simulink model "Postoian"  (R2019a)
settings: Solver=FixedStepAuto  StartTime=0.0  StopTime=1  FixedStep=0.0001  RelTol=1e-4
values from neighbouring files (symbols this model uses):
  b1 = [3.31578564644 0.905199348927 -1.07588481903 -9.39754581451 6.51989841461 -7.39431810379 -7.98054647446 -7.51470994949 -2.46217346191 -2.60606265068 0.634998142719 -7.34759140015 ... (20 elements, 1x20)]    [b1.mat]
  b2 = [-8.908867836 -6.37810707092 -8.66125679016 -6.19361543655 -8.59416675568 -9.12425804138 -8.47231483459 -9.20506572723 -8.79118919373 -9.36305236816 -9.80707740784 -1.32926535606 ... (15 elements, 1x15)]    [b2.mat]
  b3 = 0.566753208637    [b3.mat]
  w1 = [-3.38608121872 -1.61282348633 -0.811974227428 -26.1486988068 -5.43596601486 -2.50496292114 -2.73406887054 -1.47529745102 -13.9745950699 -4.77835845947 -8.42057037354 -10.048833847 ... (100 elements, 5x20)]    [w1.mat]    (also in w1d.mat = [-28.5484638214 -28.3087368011 -16.2038860321 -18.8476390839)
  w2 = [-1.73702144623 -0.185042783618 -1.43662083149 5.53469181061 0.114013127983 -6.10858488083 1.57797574997 1.2862662077 -7.84612417221 -0.614148855209 -15.9998350143 -5.41085386276 ... (300 elements, 20x15)]    [w2.mat]    (also in w2d.mat = [-15.8134098053 -19.7163829803 -21.1157608032 -0.21424435079)
  w3 = [0.296215087175 2.04968070984 0.382735908031 1.65471422672 0.95603877306]    [w3.mat]    (also in w3d.mat = [-2.66624140739 1.28664553165 0.95645904541 -5.20410871506 2)
libraries: simulink x2, neural x2
settings Model: NumberOfSteps=10  Creator=70810  LastModifiedBy=70810
settings SolverCC: AlgebraicLoopSolver=LineSearch

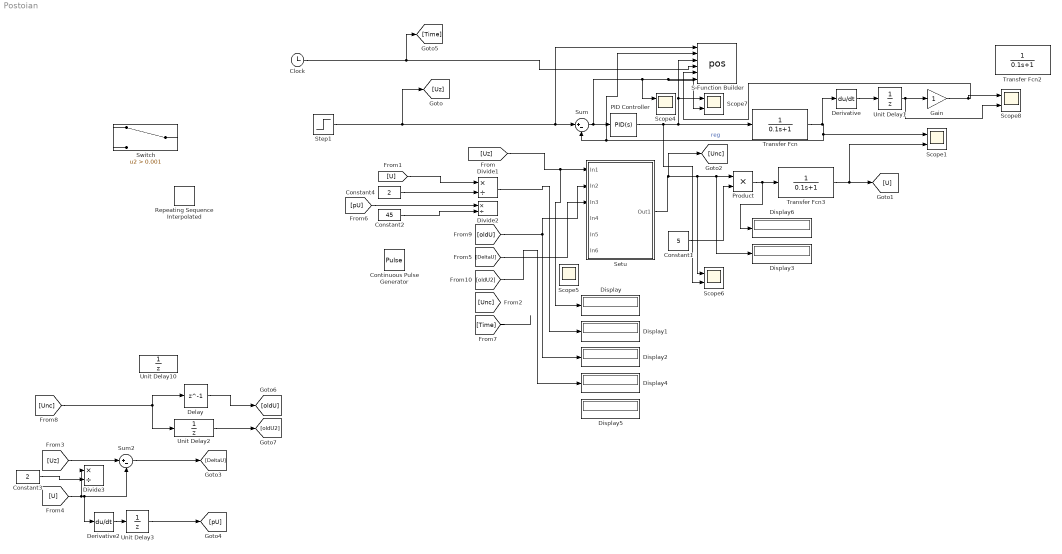
== system Postoian ==
  Clock : Clock
  Constant1 : Constant  Value=5
  Constant2 : Constant  Value=45
  Constant3 : Constant  Value=2
  Constant4 : Constant  Value=2
  Continuous Pulse Generator : DiscretePulseGenerator  PulseType=Time based  Period=1  PulseWidth=50
  Delay : Delay  DelayLength=1  InitialCondition=0
  Derivative : Derivative
  Derivative2 : Derivative
  Display{,1..6} (7 alike) : Display
  Divide1 : Product  Inputs=*/
  Divide2 : Product  Inputs=*/
  Divide3 : Product  Inputs=*/
  Gain : Gain
  PID Controller : simulink/Continuous/PID Controller  Controller=PID  Form=Parallel  TimeDomain=Continuous-time  SampleTime=-1  IntegratorMethod=Forward Euler  FilterMethod=Forward Euler  ControllerParametersSource=internal  P=4  I=255  D=0  UseFilter=on  N=100  TunerSelectOption=Transfer Function Based (PID Tuner App)  InitialConditionSource=internal  InitialConditionForIntegrator=0  InitialConditionForFilter=0  DifferentiatorICPrevScaledInput=0  ExternalReset=none  TrackingMode=off  Kt=1  LimitOutput=off  UpperSaturationLimit=inf  LowerSaturationLimit=-inf  LinearizeAsGain=on  AntiWindupMode=none  Kb=1  POutMin=[]  POutMax=[]  IOutMin=[]  IOutMax=[]  DOutMin=[]  DOutMax=[]  NOutMin=[]  NOutMax=[]  SumOutMin=[]  SumOutMax=[]  SaturationOutMin=[]  SaturationOutMax=[]  PParamMin=[]  PParamMax=[]  IParamMin=[]  IParamMax=[]  DParamMin=[]  DParamMax=[]  NParamMin=[]  NParamMax=[]  KbParamMin=[]  KbParamMax=[]  KtParamMin=[]  KtParamMax=[]  KbOutMin=[]  KbOutMax=[]  KtOutMin=[]  KtOutMax=[]  IntegratorOutMin=[]  IntegratorOutMax=[]  FilterOutMin=[]  FilterOutMax=[]  SumI1OutMin=[]  SumI1OutMax=[]  SumI2OutMin=[]  SumI2OutMax=[]  SumI3OutMin=[]  SumI3OutMax=[]  SumI4OutMin=[]  SumI4OutMax=[]  SumDOutMin=[]  SumDOutMax=[]  DifferentiatorOutMin=[]  DifferentiatorOutMax=[]  FilterDiffOutCoefMin=[]  FilterDiffOutCoefMax=[]  ReciprocalOutMin=[]  ReciprocalOutMax=[]  SumDenOutMin=[]  SumDenOutMax=[]  SumNumOutMin=[]  SumNumOutMax=[]  DivideOutMin=[]  DivideOutMax=[]  IntegratorContinuousStateAttributes=''  IntegratorStateMustResolveToSignalObject=off  IntegratorRTWStateStorageClass=Auto  FilterContinuousStateAttributes=''  FilterStateMustResolveToSignalObject=off  FilterRTWStateStorageClass=Auto  ParallelPVariant=InternalParameters  IdealPVariant=Disabled  IVariant=InternalParameters  DVariant=InternalParameters  IntegratorVariant=Continuous  SatVariant=Disabled  AWVariant=Passthrough  PCopyVariant=Disabled  TRVariant=Disabled  FdbkBlocksVariant=Forward  IdealPFdbkVariant=Disabled  SatFdbkVariant=Disabled  DerivativeFilterVariant=ContFilter  NVariant=InternalParameters  NCopyVariant=Disabled  FilterICVariant=InternalICsFilter  IntegratorICVariant=InternalICs  ExternalResetVariant=Disabled  TRSumVariant=Passthrough  SumFdbkVariant=Disabled  SumVariant=Sum_PID
  Product : Product
  Repeating Sequence Interpolated : simulink/Sources/Repeating Sequence Interpolated  OutValues=[0 0.5 1 1 0.5 0].'  TimeValues=[0 0.2 0.4 0.6 0.8 1].'  LookUpMeth=Interpolation-Use End Values  tsamp=0.01  OutMin=[]  OutMax=[]  OutDataTypeStr=double  OutputDataTypeScalingMode=double  OutDataType=fixdt(0,8)  OutScaling=2^-10
  S-Function Builder : S-Function  InitFcn=try, set_param(gcb,'FunctionName','pos'), end  FunctionName=pos  SFunctionModules=pos_wrapper Aray  SFunctionDeploymentMode=off  EnableBusSupport=off  mask(S-Function Builder){}
      mask help: Simulink:masks:SFunctionBuilder_MD
      mask init:
      | val = [[.9  0.75 0.75 1 1 .9 .9 1]',[1 1 0.75 0.75 .9 .9 1 .9]'];try , sys = get_param(gcb,'SfunBuilderFcnName');if isempty(sys), sys = get_param(gcb,'FunctionName'); end,catch, sys = get_param(gcb,'FunctionName'); end
      settings: CopyFcn=set_param(gcbh,'LinkStatus','none')  PreSaveFcn=try, set_param(gcb,'FunctionName','pos'), end  OpenFcn=sfunctionwizard(gcbh)
      mask Display: plot(val(:,1),val(:,2)),disp(sys), port_label('input',1,'u0'), port_label('input',2,'u1'), port_label('input',3,'u2'), port_label('input',4,'u3'), port_label('input',5,'u4'), port_label('input',6,'u5'), port_label('output',1,'y0')
  Scope{1,4..8} (6 alike) : Scope  NumInputPorts=2
  Setu : Subsystem
  Step1 : Step  Time=0.1  SampleTime=0
  Sum : Sum  Inputs=|+-
  Sum2 : Sum  Inputs=|+-
  Switch : Switch  Criteria=u2 > Threshold  Threshold=0.001
  Transfer Fcn : TransferFcn  Denominator=[0.1 1]
  Transfer Fcn2 : TransferFcn  Denominator=[0.1 1]
  Transfer Fcn3 : TransferFcn  Denominator=[0.1 1]
  Unit Delay1 : UnitDelay  SampleTime=0.0001  HasFrameUpgradeWarning=on
  Unit Delay10 : UnitDelay  SampleTime=0.0001  HasFrameUpgradeWarning=on
  Unit Delay2 : UnitDelay  SampleTime=0.0002  HasFrameUpgradeWarning=on
  Unit Delay3 : UnitDelay  SampleTime=0.0001  HasFrameUpgradeWarning=on
  wires:
  PID Controller/1 -> Scope6/2, Scope7/1, S-Function Builder/3, Transfer Fcn/1
  Transfer Fcn/1 -> Derivative/1, Scope1/1, Sum/2, S-Function Builder/2  "reg"
  Sum/1 -> Scope4/1, Scope7/2, S-Function Builder/6, PID Controller/1
  Product/1 -> Display6/1, Transfer Fcn3/1
  Transfer Fcn3/1 -> [U], Scope1/2
  Constant4/1 -> Divide1/2
  Constant1/1 -> Product/2
  Derivative/1 -> Unit Delay1/1
  Unit Delay1/1 -> Scope8/2, Gain/1
  Gain/1 -> Scope8/1, S-Function Builder/5
  Constant2/1 -> Divide2/2
  Step1/1 -> [Uz], S-Function Builder/1, Sum/1
  Clock/1 -> [Time], S-Function Builder/4
  [Uz] -> Sum2/1
  [U] -> Divide3/1, Sum2/2, Derivative2/1
  Sum2/1 -> [DeltaU]
  Derivative2/1 -> Unit Delay3/1
  Unit Delay3/1 -> [pU]
  [Uz] -> Display/1, Setu/1(In1)
  [U] -> Divide1/1
  [pU] -> Divide2/1
  Setu/1(Out1) -> [Unc], Scope6/1, Display3/1, Product/1
  Unit Delay2/1 -> [oldU2]
  [oldU2] -> Display4/1
  Constant3/1 -> Divide3/2
  [Unc] -> Delay/1, Unit Delay2/1
  Divide1/1 -> Display1/1
  [Time] -> ?
  [oldU] -> Setu/2(In2), Display2/1
  Delay/1 -> [oldU]
  [DeltaU] -> Setu/3(In3)

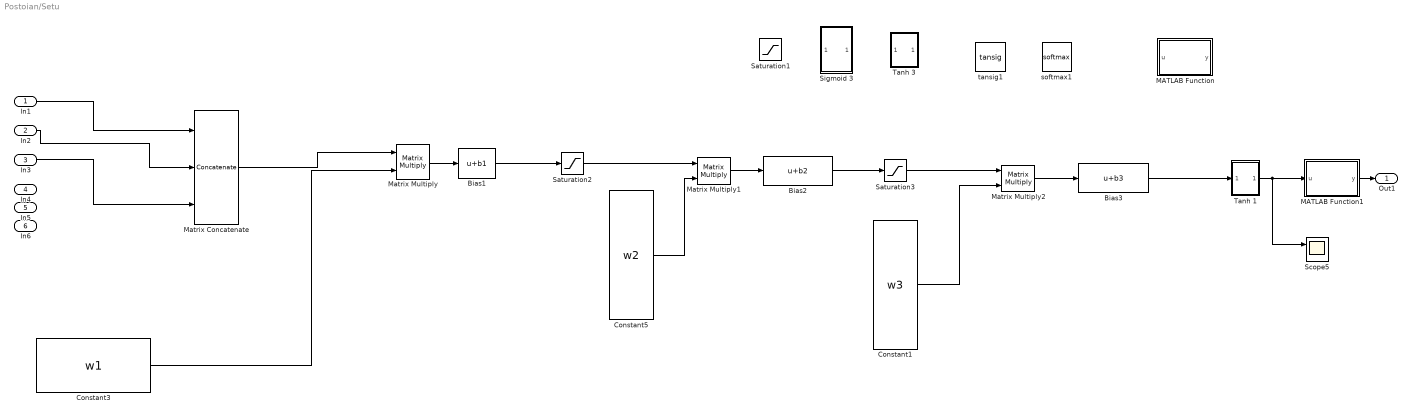
== system Postoian/Setu ==
  In1 : Inport
  In2 : Inport  Port=2
  In3 : Inport  Port=3
  In4 : Inport  Port=4
  In5 : Inport  Port=5
  In6 : Inport  Port=6
  Bias1 : Bias  Bias=b1
  Bias2 : Bias  Bias=b2
  Bias3 : Bias  Bias=b3
  Constant1 : Constant  Value=w3  VectorParams1D=off
  Constant3 : Constant  Value=w1  VectorParams1D=off
  Constant5 : Constant  Value=w2  VectorParams1D=off
  MATLAB Function : MATLAB Function  TreatAsAtomicUnit=on
  MATLAB Function1 : MATLAB Function  TreatAsAtomicUnit=on
  Matrix Concatenate : Concatenate  NumInputs=3  Mode=Multidimensional array  ConcatenateDimension=2
  Matrix Multiply : Product  Multiplication=Matrix(*)
  Matrix Multiply1 : Product  Multiplication=Matrix(*)
  Matrix Multiply2 : Product  Multiplication=Matrix(*)
  Saturation1 : Saturate  UpperLimit=inf  LowerLimit=0
  Saturation2 : Saturate  UpperLimit=inf  LowerLimit=0
  Saturation3 : Saturate  UpperLimit=inf  LowerLimit=0
  Scope5 : Scope  NumInputPorts=2
  Sigmoid 3 : Subsystem
  Tanh 1 : Subsystem
  Tanh 3 : Subsystem
  softmax1 : neural/Transfer Functions/softmax
      settings: SourceProductName=MATLAB Runtime - Deep Learning Toolbox  SourceProductBaseCode=Missing
  tansig1 : neural/Transfer Functions/tansig
      settings: SourceProductName=MATLAB Runtime - Deep Learning Toolbox  SourceProductBaseCode=Missing
  Out1 : Outport
  wires:
  Matrix Concatenate/1 -> Matrix Multiply/1
  In1/1 -> Matrix Concatenate/1
  Constant5/1 -> Matrix Multiply1/2
  In2/1 -> Matrix Concatenate/2
  Matrix Multiply1/1 -> Bias2/1
  Constant3/1 -> Matrix Multiply/2
  Matrix Multiply/1 -> Bias1/1
  Constant1/1 -> Matrix Multiply2/2
  Matrix Multiply2/1 -> Bias3/1
  Bias1/1 -> Saturation2/1
  Saturation3/1 -> Matrix Multiply2/1
  Bias3/1 -> Tanh 1/1(In1)
  Saturation2/1 -> Matrix Multiply1/1
  Tanh 1/1(Out1) -> MATLAB Function1/1(u), Scope5/1
  In3/1 -> Matrix Concatenate/3
  MATLAB Function1/1(y) -> Out1/1
  Bias2/1 -> Saturation3/1

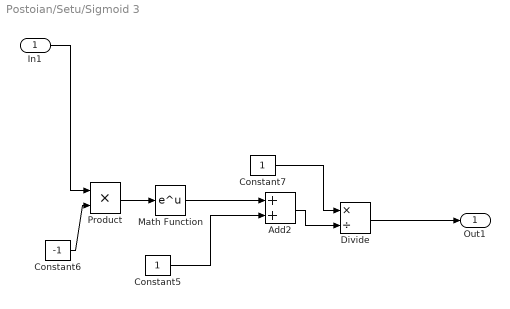
== system Postoian/Setu/Sigmoid 3 ==
  In1 : Inport
  Add2 : Sum
  Constant5 : Constant  VectorParams1D=off
  Constant6 : Constant  Value=-1  VectorParams1D=off
  Constant7 : Constant  VectorParams1D=off
  Divide : Product  Inputs=*/
  Math Function : Math  SaturateOnIntegerOverflow=on
  Product : Product
  Out1 : Outport
  wires:
  Product/1 -> Math Function/1
  Math Function/1 -> Add2/1
  Constant5/1 -> Add2/2
  Constant7/1 -> Divide/1
  Constant6/1 -> Product/2
  In1/1 -> Product/1
  Add2/1 -> Divide/2
  Divide/1 -> Out1/1

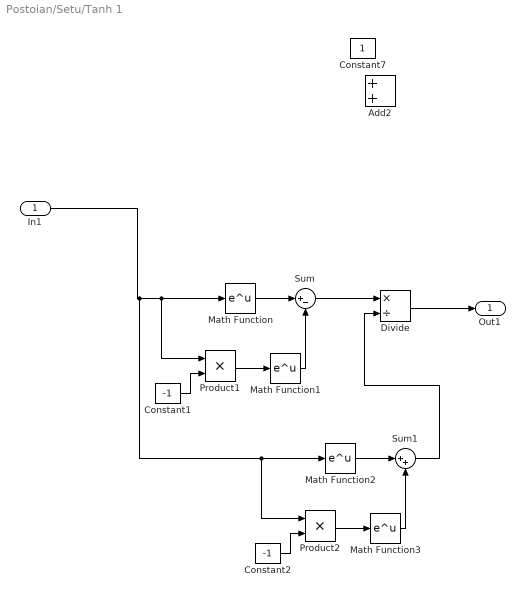
== system Postoian/Setu/Tanh 1 ==
  In1 : Inport
  Add2 : Sum
  Constant1 : Constant  Value=-1  VectorParams1D=off
  Constant2 : Constant  Value=-1  VectorParams1D=off
  Constant7 : Constant  VectorParams1D=off
  Divide : Product  Inputs=*/
  Math Function{,1..3} (4 alike) : Math  SaturateOnIntegerOverflow=on
  Product1 : Product
  Product2 : Product
  Sum : Sum  Inputs=|+-
  Sum1 : Sum  Inputs=|++
  Out1 : Outport
  wires:
  Divide/1 -> Out1/1
  Sum1/1 -> Divide/2
  Product2/1 -> Math Function3/1
  Math Function2/1 -> Sum1/1
  In1/1 -> Math Function/1, Product1/1, Math Function2/1, Product2/1
  Constant2/1 -> Product2/2
  Math Function3/1 -> Sum1/2
  Sum/1 -> Divide/1
  Math Function1/1 -> Sum/2
  Constant1/1 -> Product1/2
  Math Function/1 -> Sum/1
  Product1/1 -> Math Function1/1
  ? -> Add2/2

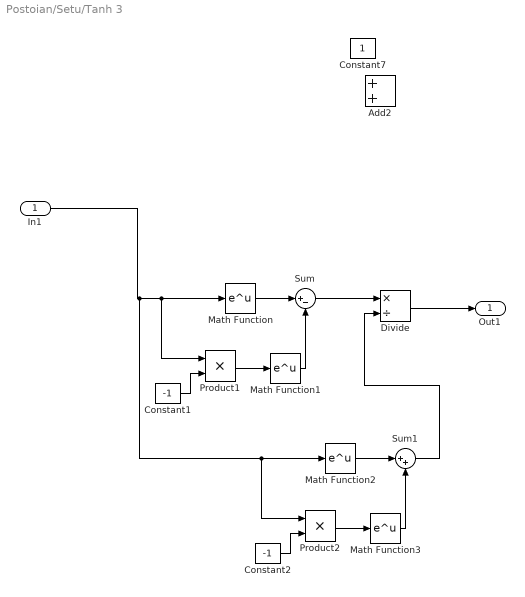
== system Postoian/Setu/Tanh 3 ==
  In1 : Inport
  Add2 : Sum
  Constant1 : Constant  Value=-1  VectorParams1D=off
  Constant2 : Constant  Value=-1  VectorParams1D=off
  Constant7 : Constant  VectorParams1D=off
  Divide : Product  Inputs=*/
  Math Function{,1..3} (4 alike) : Math  SaturateOnIntegerOverflow=on
  Product1 : Product
  Product2 : Product
  Sum : Sum  Inputs=|+-
  Sum1 : Sum  Inputs=|++
  Out1 : Outport
  wires:
  ? -> Add2/2
  Product1/1 -> Math Function1/1
  Math Function/1 -> Sum/1
  Constant1/1 -> Product1/2
  Math Function1/1 -> Sum/2
  Sum/1 -> Divide/1
  Math Function3/1 -> Sum1/2
  Constant2/1 -> Product2/2
  In1/1 -> Product2/1, Math Function2/1, Product1/1, Math Function/1
  Math Function2/1 -> Sum1/1
  Product2/1 -> Math Function3/1
  Sum1/1 -> Divide/2
  Divide/1 -> Out1/1

== matlab function Postoian/Setu/MATLAB Function1 ==
  data: u input; y output
function y = fcn(u)
if(u<0.01)
u=0;
end
y = u;

== matlab function Postoian/Setu/MATLAB Function ==
  data: u input; y output
function y = fcn(u)
if(u<0.01)
u=0;
end
y = u;
